simulink model "Step_transferfunksjon"  (R2024b)
settings: Solver=VariableStepAuto  StartTime=0.0  StopTime=0.035  RelTol=1e-3
model workspace (MATLAB code in the model file):
  | %% Step 100
  | f100 = 105;
  | wn100 = 2*pi*f100;
  | zeta100 = 1;
  | 
  | %% Step 75
  | f75 = 105;
  | wn75 = 2*pi*f75;
  | zeta75 = 0.925;
  | 
  | %% Step 50
  | f50 = 105;
  | wn50 = 2*pi*f50;
  | zeta50 = 0.925;
  | 
  | %% Step 25
  | f25 = 105;
  | wn25 = 2*pi*f25;
  | zeta25 = 0.925;
settings Model: Creator=student  LastModifiedBy=Line Kvinlaug

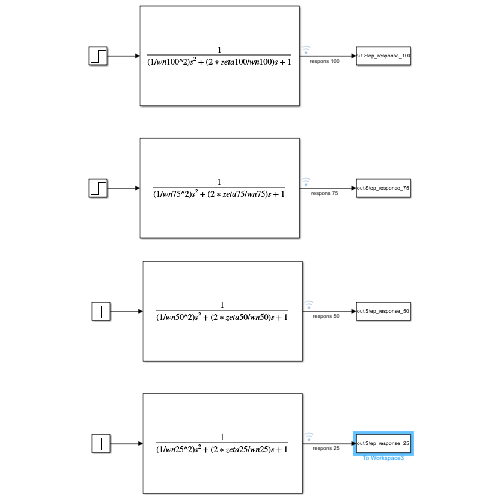
[thumbnail: Simulink's stored preview of the top-level diagram]
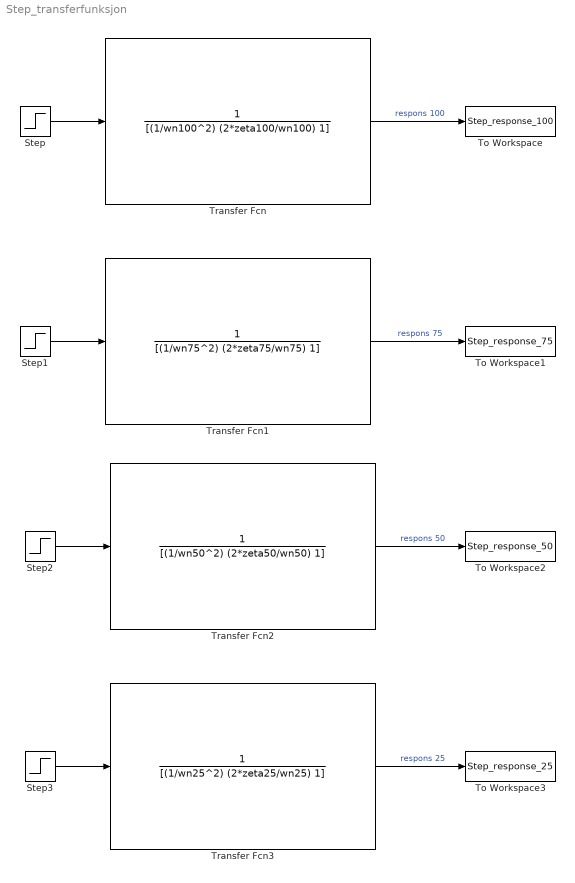
== system Step_transferfunksjon ==
  Step : Step  Time=0  After=100  SampleTime=0
  Step1 : Step  Time=0  After=75  SampleTime=0
  Step2 : Step  Time=0  After=50  SampleTime=0
  Step3 : Step  Time=0  After=25  SampleTime=0
  To Workspace : ToWorkspace  VariableName=Step_response_100  SaveFormat=Structure With Time  SampleTime=-1
  To Workspace1 : ToWorkspace  VariableName=Step_response_75  SaveFormat=Structure With Time  SampleTime=-1
  To Workspace2 : ToWorkspace  VariableName=Step_response_50  SaveFormat=Structure With Time  SampleTime=-1
  To Workspace3 : ToWorkspace  VariableName=Step_response_25  SaveFormat=Structure With Time  SampleTime=-1
  Transfer Fcn : TransferFcn  Denominator=[(1/wn100^2) (2*zeta100/wn100) 1]
  Transfer Fcn1 : TransferFcn  Denominator=[(1/wn75^2) (2*zeta75/wn75) 1]
  Transfer Fcn2 : TransferFcn  Denominator=[(1/wn50^2) (2*zeta50/wn50) 1]
  Transfer Fcn3 : TransferFcn  Denominator=[(1/wn25^2) (2*zeta25/wn25) 1]
  wires:
  Step/1 -> Transfer Fcn/1
  Transfer Fcn/1 -> To Workspace/1  "respons 100"
  Transfer Fcn1/1 -> To Workspace1/1  "respons 75"
  Step1/1 -> Transfer Fcn1/1
  Step3/1 -> Transfer Fcn3/1
  Transfer Fcn3/1 -> To Workspace3/1  "respons 25"
  Transfer Fcn2/1 -> To Workspace2/1  "respons 50"
  Step2/1 -> Transfer Fcn2/1
